simulink library "rwa_null_allocator"  (R2018b)
settings: Solver=VariableStepAuto  StartTime=0.0  StopTime=10.0  RelTol=1e-3
settings Model: Creator=Nick's PC  LastModifiedBy=Nick's PC

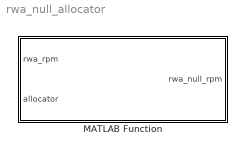
== system rwa_null_allocator ==
  MATLAB Function : MATLAB Function  TreatAsAtomicUnit=on

== matlab function rwa_null_allocator/MATLAB Function ==
  data: rwa_rpm input; rwa_null_rpm output; allocator input
function rwa_null_rpm = rwa_null_allocator(rwa_rpm, allocator)
%#codegen

RPM2RPS = 2*pi/60;
RPS2RPM = 1/RPM2RPS;

h_targ = allocator.h_targ_wheel_Nms;

nullvec = allocator.nullvec;

h_rwa = rwa_rpm .* RPM2RPS .* allocator.inertia;

h_err = h_targ - h_rwa;

h_err_null_norm = h_err ./ nullvec;

rw_max = max(h_err_null_norm);

rw_min = min(h_err_null_norm);

null_multiplier = (rw_max + rw_min)/2;

rwa_optimal_null_Nm = -null_multiplier*nullvec;

rwa_null_rpm = (rwa_optimal_null_Nm ./ allocator.inertia) .* RPS2RPM;

end
